simulink subsystem "spacing_controller"  (R2021b)
settings: Solver=VariableStepAuto  StartTime=0.0  StopTime=10.0  RelTol=1e-3
values from neighbouring files (symbols this model uses):
  C1 = 150000    [truck_trailer_model.m]
undefined symbols (not defined in the file or in its folder): L, omega, zeta
settings Model: Creator=gabep  LastModifiedBy=gabep

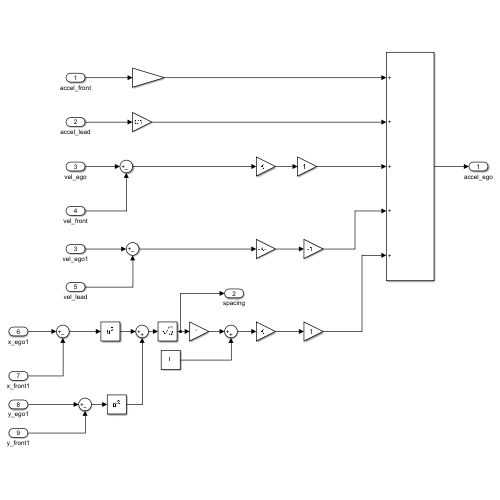
[thumbnail: Simulink's stored preview of the top-level diagram]
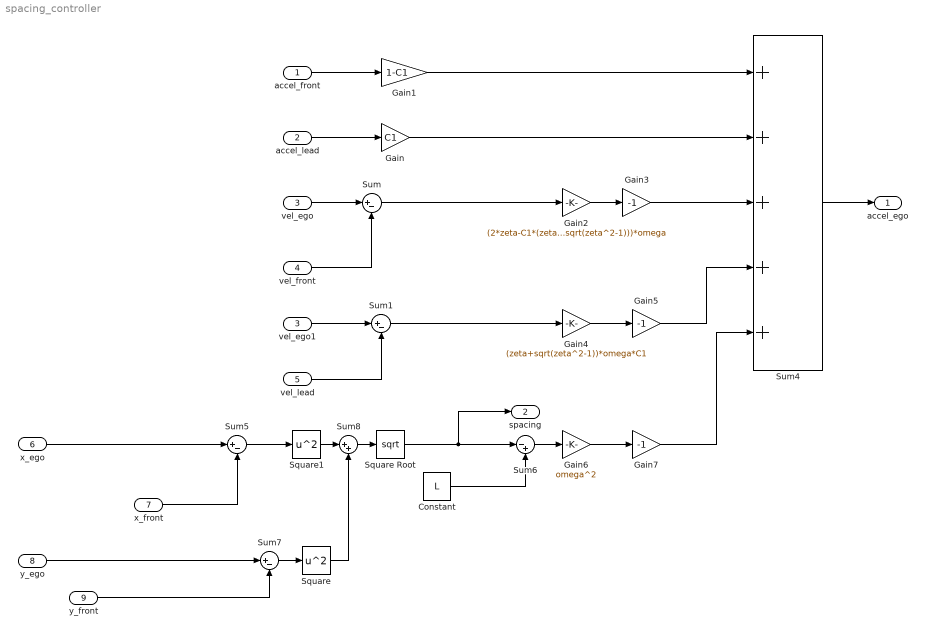
== system spacing_controller ==
  accel_front : Inport
  accel_lead : Inport  Port=2
  vel_ego : Inport  Port=3
  vel_front : Inport  Port=4
  vel_lead : Inport  Port=5
  x_ego : Inport  Port=6
  x_front : Inport  Port=7
  y_ego : Inport  Port=8
  y_front : Inport  Port=9
  Constant : Constant  Value=L
  Gain : Gain  Gain=C1
  Gain1 : Gain  Gain=1-C1
  Gain2 : Gain  Gain=(2*zeta-C1*(zeta+sqrt(zeta^2-1)))*omega
  Gain3 : Gain  Gain=-1
  Gain4 : Gain  Gain=(zeta+sqrt(zeta^2-1))*omega*C1
  Gain5 : Gain  Gain=-1
  Gain6 : Gain  Gain=omega^2
  Gain7 : Gain  Gain=-1
  Square : Math  Operator=square  SaturateOnIntegerOverflow=on
  Square Root : Sqrt  SaturateOnIntegerOverflow=on
  Square1 : Math  Operator=square  SaturateOnIntegerOverflow=on
  Sum{,1,5,7} (4 alike) : Sum  Inputs=|+-
  Sum4 : Sum  Inputs=+++++
  Sum6 : Sum  Inputs=|-+
  Sum8 : Sum  Inputs=|++
  vel_ego1 : InportShadow  Port=3
  accel_ego : Outport
  spacing : Outport  Port=2
  wires:
  accel_lead/1 -> Gain/1
  accel_front/1 -> Gain1/1
  vel_ego/1 -> Sum/1
  vel_front/1 -> Sum/2
  Sum/1 -> Gain2/1
  Gain2/1 -> Gain3/1
  vel_ego1/1 -> Sum1/1
  vel_lead/1 -> Sum1/2
  Sum1/1 -> Gain4/1
  Gain4/1 -> Gain5/1
  Gain6/1 -> Gain7/1
  Sum4/1 -> accel_ego/1
  Gain1/1 -> Sum4/1
  Gain/1 -> Sum4/2
  Gain3/1 -> Sum4/3
  Gain5/1 -> Sum4/4
  Gain7/1 -> Sum4/5
  Constant/1 -> Sum6/2
  Sum6/1 -> Gain6/1
  Sum7/1 -> Square/1
  x_front/1 -> Sum5/2
  y_ego/1 -> Sum7/1
  Square1/1 -> Sum8/1
  Sum5/1 -> Square1/1
  x_ego/1 -> Sum5/1
  Square/1 -> Sum8/2
  y_front/1 -> Sum7/2
  Square Root/1 -> spacing/1, Sum6/1
  Sum8/1 -> Square Root/1
